simulink model "invPlantSw_AFTER_SRFPLL"  (R2026a)
settings: Solver=FixedStepDiscrete  StopTime=0.15  FixedStep=ip.Ts_power
model workspace (MATLAB code in the model file):
  | ip = invParams();
libraries: fl_lib x7, nesl_utility x6, invLib x4, ee_lib x2, srfPllLib x1
settings Model: Creator=phamn  LastModifiedBy=aqiba
settings SimscapeCC: SimscapeLogType=none

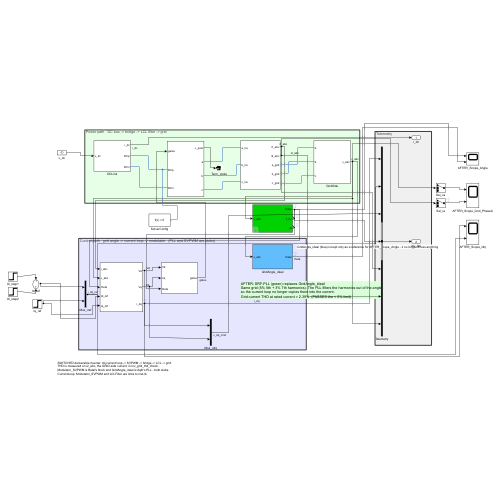
[thumbnail: Simulink's stored preview of the top-level diagram]
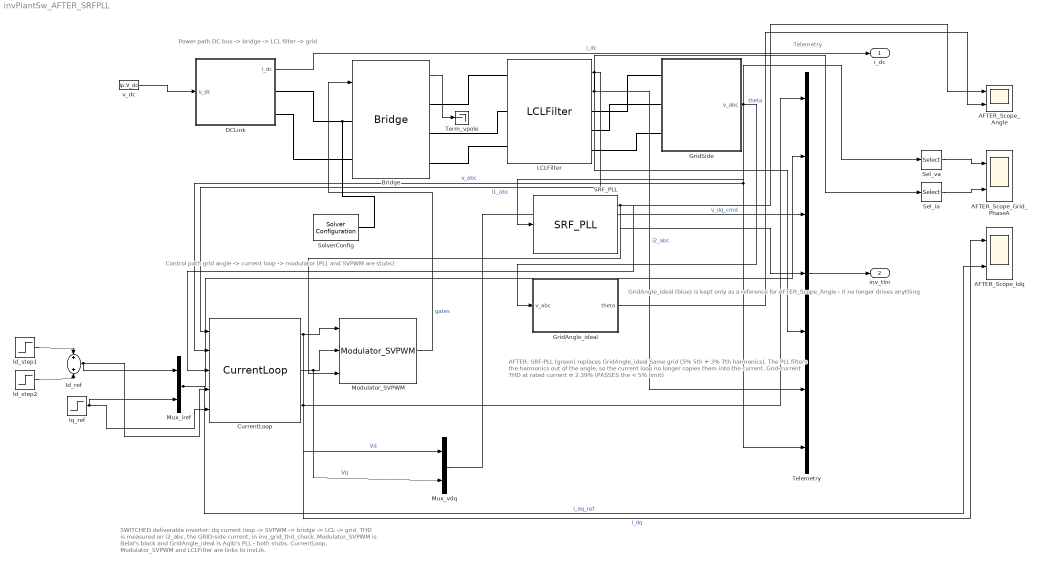
== system invPlantSw_AFTER_SRFPLL ==
  note: Power path DC bus -> bridge -> LCL filter -> grid
  note: Control path grid angle -> current loop -> modulator (PLL and SVPWM are stubs)
  note: Telemetry
  note: SWITCHED deliverable inverter: dq current loop -> SVPWM -> bridge -> LCL -> grid.
      | THD is measured on i2_abc, the GRID-side current, in inv_grid_thd_check.
      | Modulator_SVPWM is Belal's block and GridAngle_ideal is Aqib's PLL - both stubs.
      | CurrentLoop, Modulator_SVPWM and LCLFilter are links to invLib.
  note: AFTER: SRF-PLL (green) replaces GridAngle_ideal
      | Same grid (5% 5th + 3% 7th harmonics). The PLL filters the harmonics out of the angle,
      | so the current loop no longer copies them into the current.
      | Grid-current THD at rated current = 2.39%  (PASSES the < 5% limit)
  note: GridAngle_ideal (blue) is kept only as a reference for AFTER_Scope_Angle - it no longer drives anything
  AFTER_Scope_Angle : Scope  NumInputPorts=2
      settings: SampleTime=1e-5  TimeSpan=0.03  Title=AFTER (SRF-PLL): theta from SRF\_PLL (1) vs GridAngle\_ideal reference (2)  ActiveDisplayYMinimum=-3.5  ActiveDisplayYMaximum=3.5
  AFTER_Scope_Grid_PhaseA : Scope  NumInputPorts=2
      settings: SampleTime=1e-5  TimeSpan=0.03  Title=AFTER (SRF-PLL): grid voltage & grid current, phase A  ActiveDisplayYMinimum=-400  ActiveDisplayYMaximum=400
  AFTER_Scope_Idq : Scope  NumInputPorts=2
      settings: SampleTime=1e-5  Title=AFTER (SRF-PLL): Id, Iq measured vs reference  ActiveDisplayYMinimum=-60  ActiveDisplayYMaximum=360
  Bridge : invLib/Bridge  SystemSampleTime=-1  VariantActivationTime=update diagram  EmptyChoice=off  PassThrough=off  PassThroughVariantControl=(default)  EmptyChoiceVariantControl=(default)  AllowFlexibleInterface=on  Latency=0  AutoFrameSizeCalculation=off
  CurrentLoop : invLib/CurrentLoop  SystemSampleTime=-1  VariantActivationTime=update diagram  EmptyChoice=off  PassThrough=off  PassThroughVariantControl=(default)  EmptyChoiceVariantControl=(default)  AllowFlexibleInterface=on  Latency=0  AutoFrameSizeCalculation=off
  DCLink : Subsystem
  GridAngle_ideal : Subsystem
  GridSide : Subsystem
  Id_ref : Sum
  Id_step1 : Step  Time=0.08  FinalValue=0.5*ip.I_pk  SampleTime=0
  Id_step2 : Step  Time=0.10  FinalValue=0.5*ip.I_pk  SampleTime=0
  Iq_ref : Step  Time=0.16  FinalValue=0.25*ip.I_pk  SampleTime=0
  LCLFilter : invLib/LCLFilter  SystemSampleTime=-1  VariantActivationTime=update diagram  EmptyChoice=off  PassThrough=off  PassThroughVariantControl=(default)  EmptyChoiceVariantControl=(default)  AllowFlexibleInterface=on  Latency=0  AutoFrameSizeCalculation=off
  Modulator_SVPWM : invLib/Modulator_SVPWM  SystemSampleTime=-1  VariantActivationTime=update diagram  EmptyChoice=off  PassThrough=off  PassThroughVariantControl=(default)  EmptyChoiceVariantControl=(default)  AllowFlexibleInterface=on  Latency=0  AutoFrameSizeCalculation=off
  Mux_iref : Mux  Inputs=2
  Mux_vdq : Mux  Inputs=2
  SRF_PLL : srfPllLib/SRF_PLL  Ts=ip.Ts_ctrl  f0=ip.f_grid  fbw=25  zeta=0.707
  Sel_ia : Selector  InputPortWidth=3  IndexOptions=Index vector (dialog)  Indices=1  OutputSizes=1
  Sel_va : Selector  InputPortWidth=3  IndexOptions=Index vector (dialog)  Indices=1  OutputSizes=1
  SolverConfig : nesl_utility/Solver Configuration  PhysicalDomain=network_engine_domain  SubClassName=solver  LeftPortType=input  RightPortType=generic  Tones=[]  Harmonics=[]  SimulateNoise=off  Profile=off  UseLocalSampling=off  EnableSwitchedLinearOptims=on  FrequencyDomain=off  UseCCode=off  RelTol=0.001  AbsTol=0.001  MinStep=1e-09  ToWorkspace=off  RevertToSquareIcSolve=off  NumHomotopyIterations=100  PhasorMode=off  PhasorModeNumHarmonics=1  ConsistencySolver=NEWTON_XTOL_AFTER_FTOL  CanonicalOrdering=CANONICAL  OptimizeIntermediates=OPTIMIZED  IndexReductionMethod=DerivativeReplacement  DoDC=off  ResidualTolerance=1e-09  ConsistencyTolSource=GLOBAL  ConsistencyAbsTol=0.001  ConsistencyRelTol=0.001  ConsistencyTolFactor=0.001  UseLocalSolver=on  LocalSolverChoice=NE_BACKWARD_EULER_ADVANCER  ResolveIndetEquations=on  FunctionEvalNumThread=1  LocalSolverSampleTime=ip.Ts_power  DoFixedCost=off  MaxNonlinIter=3  MaxModeIter=2  ComputeImpulses=off  ImpulseIterations=2  LinearAlgebra=auto  LinearAlgebraNumThread=0  EquationFormulation=NE_TIME_EF  DelaysMemoryBudget=1024  AutomaticFiltering=on  FilteringTimeConstant=0.001  PartitionStorageMethod=AS_NEEDED  PartitionMemoryBudget=1024  PartitionMethod=ROBUST  MultibodyUseLocalSolver=off  MultibodyLocalSolverChoice=ODE1  MultibodyLocalSolverSampleTime=0.001
  Telemetry : BusCreator  Inputs=7
  Term_vpole : Terminator
  v_dc : Constant  Value=ip.V_dc
  i_dc : Outport
  inv_tlm : Outport  Port=2
  wires:
  GridSide/1(v_abc) -> CurrentLoop/2, Telemetry/7, GridAngle_ideal/1(v_abc), Sel_va/1, SRF_PLL/1  "v_abc"
  LCLFilter/1 -> CurrentLoop/1, Telemetry/5  "i1_abc"
  CurrentLoop/1 -> Modulator_SVPWM/1, Mux_vdq/1  "Vd"
  CurrentLoop/2 -> Modulator_SVPWM/2, Mux_vdq/2  "Vq"
  Modulator_SVPWM/1 -> Bridge/1  "gates"
  Bridge/1 -> Term_vpole/1
  CurrentLoop/3 -> Telemetry/1, AFTER_Scope_Idq/1  "i_dq"
  Mux_iref/1 -> Telemetry/2, AFTER_Scope_Idq/2  "i_dq_ref"
  Mux_vdq/1 -> Telemetry/3  "v_dq_cmd"
  LCLFilter/2 -> Telemetry/6, Sel_ia/1  "i2_abc"
  DCLink/1(i_dc) -> i_dc/1  "i_dc"
  Telemetry/1 -> inv_tlm/1
  v_dc/1 -> DCLink/1(v_dc)
  Id_step1/1 -> Id_ref/1
  Id_step2/1 -> Id_ref/2
  Id_ref/1 -> CurrentLoop/4, Mux_iref/1
  Iq_ref/1 -> CurrentLoop/5, Mux_iref/2
  Sel_va/1 -> AFTER_Scope_Grid_PhaseA/1
  Sel_ia/1 -> AFTER_Scope_Grid_PhaseA/2
  SRF_PLL/1 -> CurrentLoop/3, Telemetry/4, Modulator_SVPWM/3, AFTER_Scope_Angle/1
  GridAngle_ideal/1(theta) -> AFTER_Scope_Angle/2  "theta"
  connections:
  Bridge/LConn1 -- DCLink/RConn1 -- SolverConfig/RConn1
  DCLink/RConn2 -- Bridge/LConn2
  Bridge/RConn1 -- LCLFilter/LConn1
  LCLFilter/RConn1 -- GridSide/LConn1
  Bridge/RConn2 -- LCLFilter/LConn2
  LCLFilter/RConn2 -- GridSide/LConn2
  Bridge/RConn3 -- LCLFilter/LConn3
  LCLFilter/RConn3 -- GridSide/LConn3

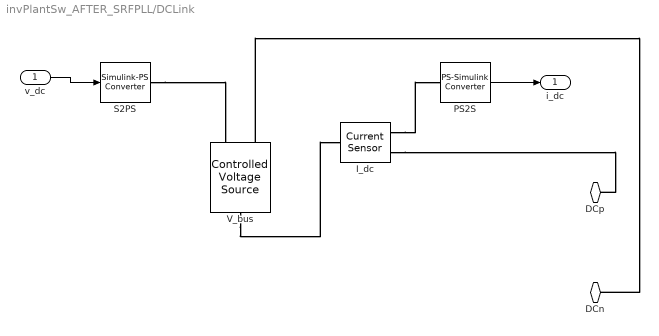
== system invPlantSw_AFTER_SRFPLL/DCLink ==
  v_dc : Inport
  I_dc : fl_lib/Electrical/Electrical Sensors/Current Sensor
  PS2S : nesl_utility/PS-Simulink Converter  PhysicalDomain=network_engine_domain  SubClassName=ps_output  LeftPortType=input  RightPortType=output  PseudoPeriodic=off  Frequencies=[]  VectorFormat=inherit  Unit=inherit  AffineConversion=off
  S2PS : nesl_utility/Simulink-PS Converter  PhysicalDomain=network_engine_domain  SubClassName=ps_input  LeftPortType=input  RightPortType=output  PseudoPeriodic=off  Frequencies=[]  NoiseDistribution=none  NoiseParameters=[]  Unit=1  AffineConversion=off  FilteringAndDerivatives=provide  SimscapeFilterOrder=1  InputFilterTimeConstant=0.001  UdotUserProvided=0
  V_bus : fl_lib/Electrical/Electrical Sources/Controlled Voltage Source
  DCp : PMIOPort  Side=Right
  DCn : PMIOPort  Port=2  Side=Right
  i_dc : Outport
  wires:
  v_dc/1 -> S2PS/1
  PS2S/1 -> i_dc/1
  connections:
  S2PS/RConn1 -- V_bus/RConn1
  V_bus/LConn1 -- I_dc/LConn1
  I_dc/RConn2 -- DCp/RConn1
  V_bus/RConn2 -- DCn/RConn1
  I_dc/RConn1 -- PS2S/LConn1

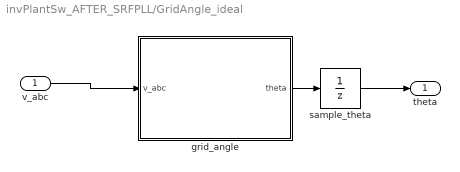
== system invPlantSw_AFTER_SRFPLL/GridAngle_ideal ==
  v_abc : Inport
  grid_angle : MATLAB Function  TreatAsAtomicUnit=on
  sample_theta : UnitDelay  SampleTime=ip.Ts_ctrl
  theta : Outport
  wires:
  v_abc/1 -> grid_angle/1(v_abc)
  grid_angle/1(theta) -> sample_theta/1
  sample_theta/1 -> theta/1

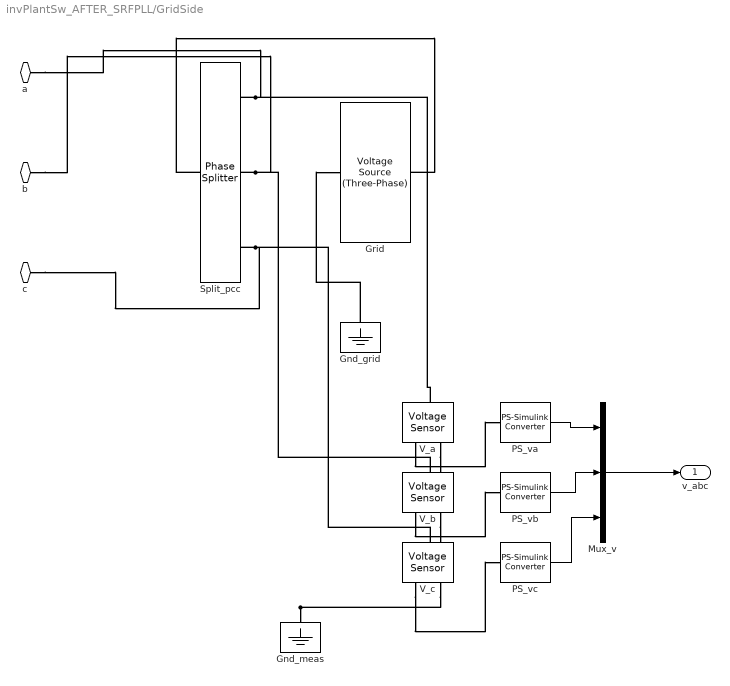
== system invPlantSw_AFTER_SRFPLL/GridSide ==
  Gnd_grid : fl_lib/Electrical/Electrical Elements/Electrical Reference
  Gnd_meas : fl_lib/Electrical/Electrical Elements/Electrical Reference
  Grid : ee_lib/Sources/Voltage Source (Three-Phase)  vline_rms=ip.V_ll V  shift=0 deg  freq=ip.f_grid Hz  impedance_option=ip.grid_Z_opt  SShortCircuit=ip.S_sc A*V  XR=ip.grid_XR  R=0.01 Ohm  L=3.97e-4 H  harmonic_option=1  harmonic_orders=[5, 7]  harmonic_ratios=[0.05, 0.03]  G_parasitic=0 1/Ohm  I_specify=off  I_priority=None  I=[0, 0, 0] A  I_nominal_specify=off  I_nominal_value=1  I_nominal_unit=A
  Mux_v : Mux  Inputs=3
  PS_va : nesl_utility/PS-Simulink Converter  PhysicalDomain=network_engine_domain  SubClassName=ps_output  LeftPortType=input  RightPortType=output  PseudoPeriodic=off  Frequencies=[]  VectorFormat=inherit  Unit=inherit  AffineConversion=off
  PS_vb : nesl_utility/PS-Simulink Converter  PhysicalDomain=network_engine_domain  SubClassName=ps_output  LeftPortType=input  RightPortType=output  PseudoPeriodic=off  Frequencies=[]  VectorFormat=inherit  Unit=inherit  AffineConversion=off
  PS_vc : nesl_utility/PS-Simulink Converter  PhysicalDomain=network_engine_domain  SubClassName=ps_output  LeftPortType=input  RightPortType=output  PseudoPeriodic=off  Frequencies=[]  VectorFormat=inherit  Unit=inherit  AffineConversion=off
  Split_pcc : ee_lib/Connectors & References/Phase Splitter
  V_a : fl_lib/Electrical/Electrical Sensors/Voltage Sensor
  V_b : fl_lib/Electrical/Electrical Sensors/Voltage Sensor
  V_c : fl_lib/Electrical/Electrical Sensors/Voltage Sensor
  a : PMIOPort  Side=Left
  b : PMIOPort  Port=2  Side=Left
  c : PMIOPort  Port=3  Side=Left
  v_abc : Outport
  wires:
  PS_va/1 -> Mux_v/1
  PS_vb/1 -> Mux_v/2
  PS_vc/1 -> Mux_v/3
  Mux_v/1 -> v_abc/1
  connections:
  Split_pcc/LConn1 -- Grid/RConn1
  Gnd_grid/LConn1 -- Grid/LConn1
  Split_pcc/RConn1 -- a/RConn1 -- V_a/LConn1
  V_a/RConn2 -- V_b/RConn2 -- Gnd_meas/LConn1 -- V_c/RConn2
  V_a/RConn1 -- PS_va/LConn1
  Split_pcc/RConn2 -- b/RConn1 -- V_b/LConn1
  V_b/RConn1 -- PS_vb/LConn1
  Split_pcc/RConn3 -- c/RConn1 -- V_c/LConn1
  V_c/RConn1 -- PS_vc/LConn1

== matlab function invPlantSw_AFTER_SRFPLL/GridAngle_ideal/grid_angle ==
  data: v_abc input; theta output
function theta = grid_angle(v_abc)
%#codegen
% Grid voltage angle straight off the Clarke transform. Not a PLL: no loop,
% no filter, no dynamics - which is the point. Aqib's SRF-PLL replaces it,
% and its lag then shows up as a difference against this baseline.
v_al = (2/3)*(v_abc(1) - 0.5*v_abc(2) - 0.5*v_abc(3));
v_be = (2/3)*(sqrt(3)/2)*(v_abc(2) - v_abc(3));
theta = atan2(v_be, v_al);
